simulink model "Quadcopter"  (R2019a)
settings: Solver=VariableStepAuto  StartTime=0.0  StopTime=2000  MaxStep=1e-1  RelTol=1e-3
StopFcn:
  | hold on;
  | plot3(out.out_y1.data, out.out_x1.data, out.out_z1.data, 'r');
  | plot3(out.out_y2.data, out.out_x2.data, out.out_z2.data, 'g');
  | plot3(out.out_y3.data, out.out_x3.data, out.out_z3.data, 'b');
  | plot3([0;out.out_y.data(1:1000:end)], [0;out.out_x.data(1:1000:end)], [0;out.out_z.data(1:1000:end)], '.k');
  | view(3);
  | hold off;
values from neighbouring files (symbols this model uses):
  B_phi = 1    [Control.m]
  B_psi = 1    [Control.m]
  B_theta = 1    [Control.m]
  B_z = 5    [Control.m]
  r_x12 = 8    [Control.m]
  r_x32 = 4    [Control.m]
  r_y12 = 8    [Control.m]
  r_y32 = 4    [Control.m]
undefined symbols (not defined in the file or in its folder): As, Bs, Cpsi, Cs, Cx, Cy, Cz, Ds, x01, x02, x03, y01, y02, y03, z01, z02, z03
libraries: simulink x1
(part 3 of 3)

== matlab function Quadcopter/scheme - double integrator/SquaDrone/Drone2/Controller/altitude ==
  data: z input; dz input; phi input; theta input; zd input; Ft output; M1 input; M2 input
function Ft = fcn(z, dz, phi, theta, zd, M1, M2)
    
    Ft = (- allf.sat(dz + allf.sat(z - zd + dz, M1), M2) + 1) / (cos(phi) * cos(theta)); 
    
end

== matlab function Quadcopter/scheme - double integrator/SquaDrone/Drone2/Controller/heading ==
  data: psid input; tau_psi output; psi input; dpsi input; M1 input; M2 input
function tau_psi = fcn(psid, psi, dpsi, M1, M2)

    tau_psi = - allf.sat(dpsi + allf.sat(psi - psid + dpsi, M1), M2);

end

== matlab function Quadcopter/scheme - double integrator/SquaDrone/Drone2/Controller/lateral ==
  data: theta input; dtheta input; thetad input; dthetad input; M1 input; tau_theta output; M2 input
function tau_theta = fcn(theta, dtheta, thetad, dthetad, M1, M2)
    
    tau_theta = - allf.sat(dtheta + allf.sat(theta - thetad + dtheta - dthetad, M1), M2);

end

== matlab function Quadcopter/single integrator/u1_x = f() ==
  data: x1 input; x2 input; x3 input; u1_x output; x_cmd input; k input; b input
function u1_x = fcn(x1, x2, x3, x_cmd, k, b)

    x_cm = (x1 + x2 + x3) / 3;
	u1_x = 3 * k * allf.sat(x_cmd - x_cm, b);
    
end

== matlab function Quadcopter/single integrator/u1_y = f() ==
  data: y1 input; y2 input; y3 input; u1_y output; y_cmd input; k input; b input
function u1_y = fcn(y1, y2, y3, y_cmd, k, b)

    y_cm = (y1 + y2 + y3) / 3;
	u1_y = 3 * k * allf.sat(y_cmd - y_cm, b);
    
end

== matlab function Quadcopter/single integrator/SquaDrone/Quadcopter1/Controller/altitude ==
  data: zd input; Ft output; z input; dz input; phi input; theta input; M1 input; M2 input
function Ft = fcn(zd, z, dz, phi, theta, M1, M2)
    
    Ft = (- allf.sat(dz + allf.sat(z - zd + dz, M1), M2) + 1) / (cos(phi) * cos(theta)); 
    
end

== matlab function Quadcopter/single integrator/SquaDrone/Quadcopter1/Controller/heading ==
  data: psid input; tau_psi output; psi input; dpsi input; M1 input; M2 input
function tau_psi = fcn(psid, psi, dpsi, M1, M2)

    tau_psi = - allf.sat(dpsi + allf.sat(psi - psid + dpsi, M1), M2);

end

== matlab function Quadcopter/single integrator/SquaDrone/Quadcopter1/Controller/lateral ==
  data: x input; dx input; theta input; dtheta input; xd input; M1 input; tau_theta output; M2 input; M3 input; M4 input
function tau_theta = fcn(x, dx, theta, dtheta, xd, M1, M2, M3, M4)
    
    z3 = dtheta + theta;
    z2 = dtheta + 2*theta - dx;
    z1 = dtheta + 3*theta - 3*dx - (x - xd);
    
    tau_theta = - allf.sat(dtheta + allf.sat(z3 + allf.sat(z2 + allf.sat(z1, M4), M3), M2), M1);

end

== matlab function Quadcopter/single integrator/SquaDrone/Quadcopter1/Controller/longitudial ==
  data: y input; dy input; phi input; dphi input; yd input; M1 input; tau_phi output; M2 input; M3 input; M4 input
function tau_phi = fcn(y, dy, phi, dphi, yd, M1, M2, M3, M4)

    z3 = dphi + phi;
    z2 = dphi + 2*phi + dy;
    z1 = dphi + 3*phi + 3*dy + y - yd;
    
    tau_phi =   - allf.sat(dphi + allf.sat(z3 + allf.sat(z2 + allf.sat(z1, M4), M3), M2), M1);

end

== matlab function Quadcopter/single integrator/SquaDrone/Quadcopter1/Dynamic_System/MATLAB Function ==
  data: Ft input; ddy output; phi input; theta input; psi input
function ddy = fcn(Ft, phi, theta, psi)
    
    ddy = Ft * cos(theta)*sin(phi);
    
end

== matlab function Quadcopter/single integrator/SquaDrone/Quadcopter1/Dynamic_System/MATLAB Function3 ==
  data: Ft input; ddx output; phi input; theta input; psi input
function ddx = fcn(Ft, phi, theta, psi)

    ddx = - Ft * sin(theta);
    
end

== matlab function Quadcopter/single integrator/SquaDrone/Quadcopter1/Dynamic_System/MATLAB Function4 ==
  data: Ft input; ddz output; phi input; theta input
function ddz = fcn(Ft, phi, theta)
    
    ddz = Ft * cos(theta)*cos(phi) - 1;
    
end

== matlab function Quadcopter/scheme - double integrator/SquaDrone/Drone2/Controller/longitudial ==
  data: phi input; dphi input; phid input; dphid input; M1 input; tau_phi output; M2 input
function tau_phi = fcn(phi, dphi, phid, dphid, M1, M2)
    
    tau_phi = - allf.sat(dphi + allf.sat(phi - phid + dphi - dphid, M1), M2);

end

== matlab function Quadcopter/scheme - double integrator/SquaDrone/Drone2/Dynamic_System/MATLAB Function ==
  data: Ft input; ddy output; phi input; theta input; psi input
function ddy = fcn(Ft, phi, theta, psi)
    
    ddy = Ft * cos(theta)*sin(phi);
    
end

== matlab function Quadcopter/scheme - double integrator/SquaDrone/Drone2/Dynamic_System/MATLAB Function3 ==
  data: Ft input; ddx output; phi input; theta input; psi input
function ddx = fcn(Ft, phi, theta, psi)

    ddx = - Ft * sin(theta);
    
end

== matlab function Quadcopter/scheme - double integrator/SquaDrone/Drone2/Dynamic_System/MATLAB Function4 ==
  data: Ft input; ddz output; phi input; theta input
function ddz = fcn(Ft, phi, theta)
    
    ddz = Ft * cos(theta)*cos(phi) - 1;
    
end

== matlab function Quadcopter/scheme - double integrator/SquaDrone/Drone3/Controller/altitude ==
  data: z input; dz input; phi input; theta input; zd input; Ft output; M1 input; M2 input
function Ft = fcn(z, dz, phi, theta, zd, M1, M2)
    
    Ft = (- allf.sat(dz + allf.sat(z - zd + dz, M1), M2) + 1) / (cos(phi) * cos(theta)); 
    
end

== matlab function Quadcopter/scheme - double integrator/SquaDrone/Drone3/Controller/heading ==
  data: psid input; tau_psi output; psi input; dpsi input; M1 input; M2 input
function tau_psi = fcn(psid, psi, dpsi, M1, M2)

    tau_psi = - allf.sat(dpsi + allf.sat(psi - psid + dpsi, M1), M2);

end

== matlab function Quadcopter/scheme - double integrator/SquaDrone/Drone3/Controller/lateral ==
  data: theta input; dtheta input; thetad input; dthetad input; M1 input; tau_theta output; M2 input
function tau_theta = fcn(theta, dtheta, thetad, dthetad, M1, M2)
    
    tau_theta = - allf.sat(dtheta + allf.sat(theta - thetad + dtheta - dthetad, M1), M2);

end

== matlab function Quadcopter/scheme - double integrator/SquaDrone/Drone3/Controller/longitudial ==
  data: phi input; dphi input; phid input; dphid input; M1 input; tau_phi output; M2 input
function tau_phi = fcn(phi, dphi, phid, dphid, M1, M2)
    
    tau_phi = - allf.sat(dphi + allf.sat(phi - phid + dphi - dphid, M1), M2);

end

== matlab function Quadcopter/scheme - double integrator/SquaDrone/Drone3/Dynamic_System/MATLAB Function ==
  data: Ft input; ddy output; phi input; theta input; psi input
function ddy = fcn(Ft, phi, theta, psi)
    
    ddy = Ft * cos(theta)*sin(phi);
    
end

== matlab function Quadcopter/scheme - double integrator/SquaDrone/Drone3/Dynamic_System/MATLAB Function3 ==
  data: Ft input; ddx output; phi input; theta input; psi input
function ddx = fcn(Ft, phi, theta, psi)

    ddx = - Ft * sin(theta);
    
end

== matlab function Quadcopter/scheme - double integrator/SquaDrone/Drone3/Dynamic_System/MATLAB Function4 ==
  data: Ft input; ddz output; phi input; theta input
function ddz = fcn(Ft, phi, theta)
    
    ddz = Ft * cos(theta)*cos(phi) - 1;
    
end

== matlab function Quadcopter/scheme - double integrator/controller x ==
  data: X_dX_ddX input; U_x output; dU_x output; X_dX_ddX_ddX_cmd input; k_b1_b2_b3 input; r input
function [U_x, dU_x] = fcn(X_dX_ddX,   X_dX_ddX_ddX_cmd, k_b1_b2_b3, r)
    

    
end

== matlab function Quadcopter/scheme - double integrator/controller y ==
  data: Y_dY_ddY input; U_Y output; dU_Y output; Y_dY_ddY_ddY_cmd input; k_b1_b2_b3 input; r input
function [U_Y, dU_Y] = fcn(Y_dY_ddY,   Y_dY_ddY_ddY_cmd, k_b1_b2_b3, r)
    

    
end

== matlab function Quadcopter/scheme - double integrator/Change input from (X,Y) to (THETA, PHI) ==
  data: U_x input; THETA_d output; dTHETA_d output; dU_x input; U_y input; dU_y input; PHI_d output; dPHI_d output
function [THETA_d, dTHETA_d, PHI_d, dPHI_d] = fcn(U_x, dU_x, U_y, dU_y)
    

    
end

== matlab function Quadcopter/double integrator/lemniscate_x ==
  data: t input; x output
function x = fcn(t)
x = sin(t) / (1 + cos(t)^2) - 1;

== matlab function Quadcopter/double integrator/lemniscate_x_derivative ==
  data: t input; dx_in output
function dx_in = fcn(t)
dx_in = cos(t)*(2 + sin(t)^2) / (1 + cos(t)^2)^2;

== matlab function Quadcopter/double integrator/lemniscate_y  ==
  data: t input; y output
function y = fcn(t)
y = sin(t)*cos(t) / (1 + cos(t)^2) - 1;

== matlab function Quadcopter/double integrator/lemniscate_y_derivative  ==
  data: t input; dy_in output
function dy_in = fcn(t)
dy_in = (cos(2*t)*(1 + cos(t)^2) + sin(2*t)*cos(t)*sin(t)) / (1 + cos(t)^2)^2;

== matlab function Quadcopter/double integrator/controller y ==
  data: y1 input; u1_y output; u2_y output; u3_y output; y2 input; y3 input; dy1 input; dy2 input; dy3 input; ddy1 input; ddy2 input; ddy3 input; y_cmd input; dy_cmd input; ddy_cmd input; dddy_cmd input; k input; b1 input; b2 input; b3 input; du1_y output; du2_y output; du3_y output; r_y12 input; r_y32 input
function [u1_y, u2_y, u3_y, du1_y, du2_y, du3_y] = fcn(y1, y2, y3, dy1, dy2, dy3, ddy1, ddy2, ddy3, y_cmd, dy_cmd, ddy_cmd, dddy_cmd, k, b1, b2, b3, r_y12, r_y32)
    
    u1_y = - (1 + k) * dy1 - k * y1 + dy2 + k * y2 - b1 * dy3 - b1 * k * y3 + b1 * ddy_cmd + b1 * (k + 1) * dy_cmd + b1 * k * y_cmd + k * r_y12;
    du1_y = - (1 + k) * ddy1 - k * dy1 + ddy2 + k * dy2 - b1 * ddy3 - b1 * k * dy3 + b1 * dddy_cmd + b1 * (k + 1) * ddy_cmd + b1 * k * dy_cmd;

    u2_y = b2 * u1_y + (b2 * k + 1) * dy1 + k * y1 - (k + 2) * dy2 - 2 * k * y2 + dy3 + k * y3 - k * r_y12 - k * r_y32;
    du2_y = b2 * du1_y + (b2 * k + 1) * ddy1 + k * dy1 - (k + 2) * ddy2 - 2 * k * dy2 + ddy3 + k * dy3;
    
    u3_y = b3*u2_y + (b3*k + 1)*dy2 + k * y2 - (k + 1)*dy3 - k*y3 + k * r_y32;
    du3_y = b3*du2_y + (b3*k + 1)*ddy2 + k * dy2 - (k + 1)*ddy3 - k*dy3;
    
end

== matlab function Quadcopter/simple system_double integrator/MATLAB Function ==
  data: x1 input; dx1 input; u1 output; x2 input; dx2 input; x3 input; dx3 input; x_cmd input; dx_cmd input; k input; b1 input; b2 input; b3 input; u2 output; u3 output; r_12 input; r_32 input
function [u1, u2, u3] = fcn(x1, dx1, x2, dx2, x3, dx3, x_cmd, dx_cmd, k, b1, b2, b3, r_12, r_32)
    
    u1 = - (1 + k) * dx1 - k * x1 + dx2 + k * x2 - b1 * dx3 - b1 * k * x3 + b1 * (k + 1) * dx_cmd + b1 * k * x_cmd + k * r_12;

    u2 = b2 * u1 + (b2 * k + 1) * dx1 + k * x1 - (k + 2) * dx2 - 2 * k * x2 + dx3 + k * x3 - k * r_12 - k * r_32;
    
    u3 = b3 * u2 + (b3*k + 1)*dx2 + k * x2 - (k + 1)*dx3 - k*x3 + k * r_32;
    
end

== matlab function Quadcopter/double integrator/controller x ==
  data: x1 input; u1_x output; u2_x output; u3_x output; x2 input; x3 input; dx1 input; dx2 input; dx3 input; ddx1 input; ddx2 input; ddx3 input; x_cmd input; dx_cmd input; ddx_cmd input; dddx_cmd input; k input; b1 input; b2 input; b3 input; du1_x output; du2_x output; du3_x output; r_x12 input; r_x32 input
function [u1_x, u2_x, u3_x, du1_x, du2_x, du3_x] = fcn(x1, x2, x3, dx1, dx2, dx3, ddx1, ddx2, ddx3, x_cmd, dx_cmd, ddx_cmd, dddx_cmd, k, b1, b2, b3, r_x12, r_x32)
    
    u1_x = - (1 + k) * dx1 - k * x1 + dx2 + k * x2 - b1 * dx3 - b1 * k * x3 + b1 * ddx_cmd + b1 * (k + 1) * dx_cmd + b1 * k * x_cmd + k * r_x12;
    du1_x = - (1 + k) * ddx1 - k * dx1 + ddx2 + k * dx2 - b1 * ddx3 - b1 * k * dx3 + b1 * dddx_cmd + b1 * (k + 1) * ddx_cmd + b1 * k * dx_cmd;

    u2_x = b2 * u1_x + (b2 * k + 1) * dx1 + k * x1 - (k + 2) * dx2 - 2 * k * x2 + dx3 + k * x3 - k * r_x12 - k * r_x32;
    du2_x = b2 * du1_x + (b2 * k + 1) * ddx1 + k * dx1 - (k + 2) * ddx2 - 2 * k * dx2 + ddx3 + k * dx3;
    
    u3_x = b3*u2_x + (b3*k + 1)*dx2 + k * x2 - (k + 1)*dx3 - k*x3 + k * r_x32;
    du3_x = b3*du2_x + (b3*k + 1)*ddx2 + k * dx2 - (k + 1)*ddx3 - k*dx3;
    
end

== matlab function Quadcopter/Quadcopter control zd, psid, thetad, phid/Controller/altitude ==
  data: z input; dz input; phi input; theta input; zd input; Ft output; M1 input; M2 input
function Ft = fcn(z, dz, phi, theta, zd, M1, M2)
    
    Ft = (- allf.sat(dz + allf.sat(z - zd + dz, M1), M2) + 1) / (cos(phi) * cos(theta)); 
    
end

== matlab function Quadcopter/Quadcopter control zd, psid, thetad, phid/Controller/heading ==
  data: psid input; tau_psi output; psi input; dpsi input; M1 input; M2 input
function tau_psi = fcn(psid, psi, dpsi, M1, M2)

    tau_psi = - allf.sat(dpsi + allf.sat(psi - psid + dpsi, M1), M2);

end

== matlab function Quadcopter/Quadcopter control zd, psid, thetad, phid/Controller/lateral ==
  data: theta input; dtheta input; thetad input; dthetad input; M1 input; tau_theta output; M2 input
function tau_theta = fcn(theta, dtheta, thetad, dthetad, M1, M2)
    
    tau_theta = - allf.sat(dtheta - dthetad + allf.sat(theta - thetad + dtheta - dthetad, M1), M2);

end

== matlab function Quadcopter/Quadcopter control zd, psid, thetad, phid/Controller/longitudial ==
  data: phi input; dphi input; phid input; dphid input; M1 input; tau_phi output; M2 input
function tau_phi = fcn(phi, dphi, phid, dphid, M1, M2)
    
    tau_phi = - allf.sat(dphi - dphid + allf.sat(phi - phid + dphi - dphid, M1), M2);

end

== matlab function Quadcopter/Quadcopter control zd, psid, thetad, phid/Dynamic_System/MATLAB Function ==
  data: Ft input; ddy output; phi input; theta input; psi input
function ddy = fcn(Ft, phi, theta, psi)
    
    ddy = Ft * cos(theta)*sin(phi);
    
end

== matlab function Quadcopter/Quadcopter control zd, psid, thetad, phid/Dynamic_System/MATLAB Function3 ==
  data: Ft input; ddx output; phi input; theta input; psi input
function ddx = fcn(Ft, phi, theta, psi)

    ddx = - Ft * sin(theta);
    
end

== matlab function Quadcopter/Quadcopter control zd, psid, thetad, phid/Dynamic_System/MATLAB Function4 ==
  data: Ft input; ddz output; phi input; theta input
function ddz = fcn(Ft, phi, theta)
    
    ddz = Ft * cos(theta)*cos(phi) - 1;
    
end
